simulink library "carnot"  (R2018b)
settings: Solver=VariableStepAuto  StartTime=0.0  StopTime=10.0  RelTol=1e-3
undefined symbols (not defined in the file or in its folder): A, A_earth, acol, Acol, ActPower1, ActPower2, ActPower3, Ad, Ad0, Ar, Au, Au0, Azimuth_Angle, B, Bd, Bd0, Br, Bu, Bu0, C, c1, c2, c3, c33, c4, c5, c6, CarnotCallbacks_Density, CarnotCallbacks_Enthalpy, CarnotCallbacks_Enthalpy2Temperature, CarnotCallbacks_Entropy, CarnotCallbacks_Evaporation_Enthalpy, CarnotCallbacks_GlobalMessageLevel, CarnotCallbacks_Grashof, CarnotCallbacks_Heat_Capacity, CarnotCallbacks_Kinematic_Viscosity, CarnotCallbacks_PMV_PPD, CarnotCallbacks_Prandtl, CarnotCallbacks_Saturation_Property, CarnotCallbacks_Saturation_Temperature, CarnotCallbacks_Saturation_Value_Water, CarnotCallbacks_Specific_Volume, CarnotCallbacks_Thermal_Conductivity, CarnotCallbacks_Vapour_Content, CarnotCallbacks_Vapour_Pressure, Cd, Cdl, Cr, Cu, Davies, Dd, DE_TRY2010_04_averageYear, delta_grd, density, DiameterLastPiece, dl, DPConstant, DPLinear, DPQuadratic, Dr ... (+59)
libraries: $bdroot x429, simulink x36, simulink_extras x12
(part 18 of 22)

== system carnot/Storage/Thermal/Storage_Ports ==
  Electric_Heating : Subsystem  mask(electric heating){hin=0.6, hout=0.65, nodes=nodes}
      mask prompts: hin "relative height start heating zone"; hout "relative height end heating zone"; nodes "Number of nodes (do not change here)"
      mask help: The block is an electric backup heating for the storage. Give inlet- and outlet-height as a relative position from 0 (= bottom) to 1 (= top).
      mask init:
      | hin = min(1, max(0, hin));
      | hout = min(1, max(0, hout));
      | 
      | if hin < hout
      |     inlet = max(ceil(hin*nodes),1);    % start node of heated zone
      |     outlet = max(ceil(hout*nodes),1);  % end node of heated zone
      | else
      |     outlet = max(ceil(hin*nodes),1);   % end node of heated zone
      |     inlet = max(ceil(hout*nodes),1);   % start node of heated zone
      | end
      | 
      | Q = zeros(nodes,1);                    % initilize power vector
      | if inlet < outlet
      |     Q(inlet:outlet) = ones(outlet-inlet+1,1); % set heated zone to One
      | else
      |     Q(outlet:inlet) = ones(inlet-outlet+1,1); % set heated zone to One
      | end
      | Q = Q./sum(Q);                         % sum over all elements must be one
      mask Help: web(fullfile(path_carnot('help'),'Electric_Heating.html'),'-helpbrowser')
      mask DialogControl ParameterTabVar0 Prompt: Geometry
      mask DialogControl ParameterTabVar01 Prompt: Top Mask Params
  HX_EN12977 : Subsystem  mask(heat exchanger for storage, data EN 12977){h_in=1, h_out=0, hgt=1, dia=0.03, height=-1, ua0=100, uam=0.1, uat=0.5, uat2=0, dplin=100, dpqua=100, nodes=nodes}
      mask prompts: h_in "relative height of inlet"; h_out "relative height of outlet"; hgt "Height of storage in m"; dia "Diameter of HX pipe [m]"; height "Height difference inlet-outlet [m]"; ua0 "uac: heat transfer coefficient [W/K /(kg/s) /(°C)]"; uam "uam: massflow dependent heat transfer [-]"; uat "uat: temperature dependent heat transfer [-]"; uat2 "uat2: temperature difference dependent heat transfer [-]"; dplin "Pressure drop coefficient dplin [Pa/(kg/s)]"; dpqua "Pressure drop coefficient dpqua [Pa/(kg/s)²]"; nodes "number of nodes"
      mask help:
      | The block transforms the incoming THV vector to a vector which the storage interprets as a heat exchanger.
      | Give inlet and outlet as a relative position 0=bottom to 1=top
      | The heat transfer is calculated by:
      | UA = uac * mdot^uam *
      |           ((Theatexchanger+Tstorage)/2)^uat *
      |           (Theatexchanger-Tstorage)^uat2
      mask init:
      | in = zeros(nodes,1);    % vector of length nodes
      | up = in;                % vector of length nodes
      | down = in;              % vector of length nodes
      | 
      | h_in = max(0,h_in);     % no nodes below 0
      | h_out = max(0,h_out);   % no nodes below 0
      | 
      | inlet = round(h_in*(nodes-1))+1;    % inlet position
      | outlet = round(h_out*(nodes-1))+1;  % outlet position
      | set_param(gcb,'height',num2str((h_out-h_in)*hgt));
      | % hgt = (h_out-h_in)*hgt;
      | 
      | in(inlet)=1;
      | 
      | if (h_in < h_out)           % if inlet below outlet
      |     up(inlet:outlet)=1;     % upwards
      | elseif (h_in > h_out)       % else if inlet above outlet
      |     down(outlet:inlet)=1;   % downwards
      | end
      mask Help: web(['file:///' fullfile(path_carnot('help'),'StoragePorts_HeatExchangerModels.html')],'-helpbrowser')
      mask TypeOptions dia: Pressure_Drop_StorageHX/dia
      mask TypeOptions height: Pressure_Drop_StorageHX/hgt
      mask TypeOptions ua0: sfun_storage_heatexchanger/p1
      mask TypeOptions uam: sfun_storage_heatexchanger/p2
      mask TypeOptions uat: sfun_storage_heatexchanger/p3
      mask TypeOptions uat2: sfun_storage_heatexchanger/p4
      mask TypeOptions dplin: Pressure_Drop_StorageHX/dplin
      mask TypeOptions dpqua: Pressure_Drop_StorageHX/dpqua
      mask TypeOptions nodes: sfun_storage_heatexchanger/nodes
      mask DialogControl ParameterTabVar0 Prompt: Geometry
      mask DialogControl ParameterTabVar01 Prompt: Heat transfer
      mask DialogControl ParameterTabVar012 Prompt: Pressure drop
      mask DialogControl ParameterTabVar0123 Prompt: Calculation
      mask Display: disp('HX EN12977')
  HX_EN12977_stratified : Subsystem  mask(stratified heat exchanger for storage, data EN 12977){h_in=1, h_out=0, hgt=height, dia=0.03, height=, ua0=100, uam=0.1, uat=0.5, uat2=0, dplin=100, dpqua=100, nodes=10}
      mask prompts: h_in "relative height of inlet"; h_out "relative height of outlet"; hgt "Height of storage in m"; dia "Diameter of HX pipe [m]"; height "Height difference inlet-outlet [m]"; ua0 "uac: heat transfer coefficient [W/K /(kg/s) /(°C)]"; uam "uam: massflow dependent heat transfer [-]"; uat "uat: temperature dependent heat transfer [-]"; uat2 "uat2: temperature difference dependent heat transfer [-]"; dplin "Pressure drop coefficient dplin [Pa/(kg/s)]"; dpqua "Pressure drop coefficient dpqua [Pa/(kg/s)²]"; nodes "number of nodes"
      mask help:
      | The block transforms the incoming THV vector to a vector which the storage interprets as a heat exchanger.
      | Give inlet and outlet as a relative position 0=bottom to 1=top
      | The heat transfer is calculated by:
      | UA = uac * mdot^uam *
      |           ((Theatexchanger+Tstorage)/2)^uat *
      |           (Theatexchanger-Tstorage)^uat2
      | Stratified:
      | For charging (inlet above outlet) the heat transfer starts when the storage temperature is below the heat exchanger temperature.
      | For discharging (outlet above inlet) the heat transfer starts when the storage temperature is above the heat exchanger temperature.
      mask init: same as carnot/Storage/Thermal/Storage_Ports/HX_EN12977
      mask Help: web(['file:///' fullfile(path_carnot('help'),'StoragePorts_HeatExchangerModels.html')],'-helpbrowser')
      mask TypeOptions dia: Pressure_Drop_StorageHX/dia
      mask TypeOptions height: Pressure_Drop_StorageHX/hgt
      mask TypeOptions ua0: sfun_storage_heatexchanger/p1
      mask TypeOptions uam: sfun_storage_heatexchanger/p2
      mask TypeOptions uat: sfun_storage_heatexchanger/p3
      mask TypeOptions uat2: sfun_storage_heatexchanger/p4
      mask TypeOptions dplin: Pressure_Drop_StorageHX/dplin
      mask TypeOptions dpqua: Pressure_Drop_StorageHX/dpqua
      mask TypeOptions nodes: sfun_storage_heatexchanger/nodes
      mask DialogControl ParameterTabVar0 Prompt: Geometry
      mask DialogControl ParameterTabVar01 Prompt: Heat transfer
      mask DialogControl ParameterTabVar012 Prompt: Pressure drop
      mask DialogControl ParameterTabVar0123 Prompt: Calculation
      mask Display: disp('HX EN12977 STRAT')
  HX_data_fit : Subsystem  mask(heat exchanger for storage, fitted data){h_in=1, h_out=0, hgt=1, dia=0.03, height=-1, ua0=100, uam=0, uat=0, dplin=10, dpqua=10, nodes=10}
      mask prompts: h_in "relative height of inlet"; h_out "relative height of outlet"; hgt "Height of storage in m"; dia "Diameter of HX pipe [m]"; height "Height difference inlet-outlet [m]"; ua0 "uac: constant heat transfer coefficient [W/K]"; uam "uam: massflow dependent heat transfer [W*s/(K*kg)]"; uat "uat: temperature difference dependent heat transfer [W/K²]"; dplin "Pressure drop coefficient dplin [Pa/(kg/s)]"; dpqua "Pressure drop coefficient dpqua [Pa/(kg/s)²]"; nodes "Number of nodes"
      mask help:
      | The block transforms the incoming THV vector to a vector which the storage interprets as a heat exchanger.
      | Give inlet and outlet as a relative position 0=bottom to 1=top
      | The heat transfer is calculated by:
      | UA = uac + mdot*uam + (Theatexchanger-Tstorage)*uat
      mask init:
      | in = zeros(nodes,1);    % vector of length nodes
      | up = in;                % vector of length nodes
      | down = in;              % vector of length nodes
      | 
      | h_in = max(0,h_in);     % no nodes below 0
      | h_out = max(0,h_out);   % no nodes below 0
      | 
      | inlet = round(h_in*(nodes-1))+1;    % inlet position
      | outlet = round(h_out*(nodes-1))+1;  % outlet position
      | set_param(gcb,'height',num2str((h_out-h_in)*hgt));
      | in(inlet)=1;
      | 
      | if (h_in < h_out)           % if inlet below outlet
      |     up(inlet:outlet)=1;     % upwards
      | elseif (h_in > h_out)       % else if inlet above outlet
      |     down(outlet:inlet)=1;   % downwards
      | end
      mask Help: web(fullfile(path_carnot('help'),'StoragePorts_HeatExchangerModels.html'),'-helpbrowser')
      mask TypeOptions dia: Pressure_Drop_StorageHX/dia
      mask TypeOptions height: Pressure_Drop_StorageHX/hgt
      mask TypeOptions ua0: sfun_storage_heatexchanger/p1
      mask TypeOptions uam: sfun_storage_heatexchanger/p2
      mask TypeOptions uat: sfun_storage_heatexchanger/p3
      mask TypeOptions dplin: Pressure_Drop_StorageHX/dplin
      mask TypeOptions dpqua: Pressure_Drop_StorageHX/dpqua
      mask TypeOptions nodes: sfun_storage_heatexchanger/nodes
      mask DialogControl ParameterTabVar0 Prompt: Geometry
      mask DialogControl ParameterTabVar01 Prompt: Heat transfer
      mask DialogControl ParameterTabVar012 Prompt: Pressure drop
      mask DialogControl ParameterTabVar0123 Prompt: Calculation
      mask Display: disp('HX data')
  HX_data_fit_stratified : Subsystem  mask(stratified heat exchanger for storage, fitted data){h_in=1, h_out=0, hgt=1.5, dia=0.03, height=-1.5, ua0=800, uam=0, uat=0, dplin=100, dpqua=100, nodes=10}
      mask prompts: h_in "relative height of inlet"; h_out "relative height of outlet"; hgt "Height of storage in m"; dia "Diameter of HX pipe [m]"; height "Height difference inlet-outlet [m]"; ua0 "uac: constant heat transfer coefficient [W/K]"; uam "uam: massflow dependent heat transfer [W*s/(K*kg)]"; uat "uat: temperature difference dependent heat transfer [W/K²]"; dplin "Pressure drop coefficient dplin [Pa/(kg/s)]"; dpqua "Pressure drop coefficient dpqua [Pa/(kg/s)²]"; nodes "number of nodes"
      mask help:
      | The block transforms the incoming THV vector to a vector which the storage interprets as a heat exchanger.
      | Give inlet and outlet as a relative position 0=bottom to 1=top
      | The heat transfer is calculated by:
      | UA = uac + mdot*uam + (Theatexchanger-Tstorage)*uat
      |
      | Stratified:
      | For charging (inlet above outlet) the heat transfer starts when the storage temperature is below the heat exchanger temperature.
      | For discharging (outlet above inlet) the heat transfer starts when the storage temperature is above the heat exchanger temperature.
      mask init: same as carnot/Storage/Thermal/Storage_Ports/HX_EN12977
      mask Help: web(['file:///' fullfile(path_carnot('help'),'StoragePorts_HeatExchangerModels.html')],'-helpbrowser')
      mask TypeOptions dia: Pressure_Drop_StorageHX/dia
      mask TypeOptions height: Pressure_Drop_StorageHX/hgt
      mask TypeOptions ua0: sfun_storage_heatexchanger/p1
      mask TypeOptions uam: sfun_storage_heatexchanger/p2
      mask TypeOptions uat: sfun_storage_heatexchanger/p3
      mask TypeOptions dplin: Pressure_Drop_StorageHX/dplin
      mask TypeOptions dpqua: Pressure_Drop_StorageHX/dpqua
      mask TypeOptions nodes: sfun_storage_heatexchanger/nodes
      mask DialogControl ParameterTabVar0 Prompt: Geometry
      mask DialogControl ParameterTabVar01 Prompt: Heat transfer
      mask DialogControl ParameterTabVar012 Prompt: Pressure drop
      mask DialogControl ParameterTabVar0123 Prompt: Calculation
      mask Display: disp('HX data STRAT')
  HX_finned_tube : Subsystem  mask(finned tube heat exchanger for storage){h_in=0.5, h_out=0, hgt=1, dpipe=0.03, swall=0.001, lpipe=10, cond=50, dfin=0.05, sfin=0.002, nfin=100, height=-0.5, dplin=100, dpqua=100, nodes=10}
      mask prompts: h_in "relative height of inlet"; h_out "relative height of outlet"; hgt "Height of storage in m"; dpipe "outer diameter of HX pipe in m (without fins)"; swall "thickness of pipe wall in m"; lpipe "length of HX pipe in m"; cond "thermal conductivity of HX wall in W/m/K"; dfin "diameter of HX pipe with fins in m"; sfin "wall thickness of fins in m"; nfin "number of fins per length in 1/m"; height "Height difference inlet-outlet [m]"; dplin "Pressure drop coefficient dplin [Pa/(kg/s)]"; dpqua "Pressure drop coefficient dpqua [Pa/(kg/s)²]"; nodes "number of nodes"
      mask help:
      | The block transforms the incoming THV vector to a vector which the storage interprets as a heat exchanger.
      | Give inlet and outlet as a relative position 0=bottom to 1=top
      | The heat transfer is calculated by a theoretical equation from Wagner: Waermeuebertragung, Vogel Fachbuch, 1991
      mask init:
      | in = zeros(nodes,1);    % vector of length nodes
      | up = in;                % vector of length nodes
      | down = in;              % vector of length nodes
      | 
      | h_in = max(0,h_in);     % no nodes below 0
      | h_out = max(0,h_out);   % no nodes below 0
      | set_param(gcb,'height',num2str((h_out-h_in)*hgt));
      | % hgt = (h_out-h_in)*hgt;
      | 
      | inlet = round(h_in*(nodes-1))+1;    % inlet position
      | outlet = round(h_out*(nodes-1))+1;  % outlet position
      | 
      | in(inlet)=1;
      | 
      | if (h_in < h_out)           % if inlet below outlet
      |     up(inlet:outlet)=1;     % upwards
      | elseif (h_in > h_out)       % else if inlet above outlet
      |     down(outlet:inlet)=1;   % downwards
      | end
      | 
      | dfin = max(dfin,dpipe);
      | nfin = max(nfin, 0);
      | if (sfin < 1e-5)
      |    sfin = 1e-5;
      |    disp('fin width set to minimum 0.01 mm')
      | end
      mask Help: web(['file:///' fullfile(path_carnot('help'),'StoragePorts_HeatExchangerModels.html')],'-helpbrowser')
      mask TypeOptions dpipe: sfun_storage_heatexchanger/p1 | Pressure_Drop_StorageHX/dia
      mask TypeOptions swall: sfun_storage_heatexchanger/p2
      mask TypeOptions lpipe: sfun_storage_heatexchanger/p3
      mask TypeOptions cond: sfun_storage_heatexchanger/p4
      mask TypeOptions dfin: sfun_storage_heatexchanger/p5
      mask TypeOptions sfin: sfun_storage_heatexchanger/p6
      mask TypeOptions nfin: sfun_storage_heatexchanger/p7
      mask TypeOptions height: Pressure_Drop_StorageHX/hgt
      mask TypeOptions dplin: Pressure_Drop_StorageHX/dplin
      mask TypeOptions dpqua: Pressure_Drop_StorageHX/dpqua
      mask TypeOptions nodes: sfun_storage_heatexchanger/nodes
      mask DialogControl ParameterTabVar0 Prompt: Heat Exchanger
      mask DialogControl ParameterTabVar01 Prompt: Pressure drop
      mask DialogControl ParameterTabVar012 Prompt: Calculation
      mask Display: disp('HX finned tube')
  HX_finned_tube_stratified : Subsystem  mask(finned tube heat exchanger for storage){h_in=1, h_out=0, hgt=1, dpipe=0.03, swall=0.001, lpipe=10, cond=50, dfin=0.05, sfin=0.002, nfin=100, height=-1, dplin=100, dpqua=100, nodes=10}
      mask prompts: h_in "relative height of inlet"; h_out "relative height of outlet"; hgt "Height of storage in m"; dpipe "outer diameter of HX pipe in m (without fins)"; swall "thickness of pipe wall in m"; lpipe "length of HX pipe in m"; cond "thermal conductivity of HX wall in W/m/K"; dfin "diameter of HX pipe with fins in m"; sfin "wall thickness of fins in m"; nfin "number of fins per length in 1/m"; height "Height difference inlet-outlet [m]"; dplin "Pressure drop coefficient dplin [Pa/(kg/s)]"; dpqua "Pressure drop coefficient dpqua [Pa/(kg/s)²]"; nodes "number of nodes"
      mask help:
      | The block transforms the incoming THV vector to a vector which the storage interprets as a heat exchanger.
      | Give inlet and outlet as a relative position 0=bottom to 1=top
      | The heat transfer is calculated by a theoretical equation from Wagner: Waermeuebertragung, Vogel Fachbuch, 1991
      mask init: same as carnot/Storage/Thermal/Storage_Ports/HX_finned_tube
      mask Help: web(['file:///' fullfile(path_carnot('help'),'StoragePorts_HeatExchangerModels.html')],'-helpbrowser')
      mask TypeOptions dpipe: sfun_storage_heatexchanger/p1 | Pressure_Drop_StorageHX/dia
      mask TypeOptions swall: sfun_storage_heatexchanger/p2
      mask TypeOptions lpipe: sfun_storage_heatexchanger/p3
      mask TypeOptions cond: sfun_storage_heatexchanger/p4
      mask TypeOptions dfin: sfun_storage_heatexchanger/p5
      mask TypeOptions sfin: sfun_storage_heatexchanger/p6
      mask TypeOptions nfin: sfun_storage_heatexchanger/p7
      mask TypeOptions height: Pressure_Drop_StorageHX/hgt
      mask TypeOptions dplin: Pressure_Drop_StorageHX/dplin
      mask TypeOptions dpqua: Pressure_Drop_StorageHX/dpqua
      mask TypeOptions nodes: sfun_storage_heatexchanger/nodes
      mask DialogControl ParameterTabVar0 Prompt: Heat Exchanger
      mask DialogControl ParameterTabVar01 Prompt: Pressure drop
      mask DialogControl ParameterTabVar012 Prompt: Calculation
      mask Display: disp('HX finned tube STRAT')
  HX_tube : Subsystem  mask(smooth tube heat exchanger for storage){h_in=0.5, h_out=0, hgt=1.5, dpipe=0.03, swall=0.001, lpipe=10, cond=50, height=-0.75, dplin=100, dpqua=100, nodes=10}
      mask prompts: h_in "relative height of inlet"; h_out "relative height of outlet"; hgt "Height of storage in m"; dpipe "outer diameter of HX pipe in m"; swall "thickness of pipe wall in m"; lpipe "length of HX pipe in m"; cond "thermal conductivity of HX wall in W/m/K"; height "Height difference inlet-outlet [m]"; dplin "Pressure drop coefficient dplin [Pa/(kg/s)]"; dpqua "Pressure drop coefficient dpqua [Pa/(kg/s)²]"; nodes "number of nodes"
      mask help:
      | The block transforms the incoming THV vector to a vector which the storage interprets as a heat exchanger.
      | Give inlet and outlet as a relative position 0=bottom to 1=top
      | The heat transfer is calculated with an equation from Wagner: Waermeuebertragung, Vogel-Verlag, 1991
      mask init: same as carnot/Storage/Thermal/Storage_Ports/HX_EN12977
      mask Help: web(['file:///' fullfile(path_carnot('help'),'StoragePorts_HeatExchangerModels.html')],'-helpbrowser')
      mask TypeOptions dpipe: sfun_storage_heatexchanger/p1
      mask TypeOptions swall: sfun_storage_heatexchanger/p2
      mask TypeOptions lpipe: sfun_storage_heatexchanger/p3
      mask TypeOptions cond: sfun_storage_heatexchanger/p4
      mask TypeOptions height: Pressure_Drop_StorageHX/hgt
      mask TypeOptions dplin: Pressure_Drop_StorageHX/dplin
      mask TypeOptions dpqua: Pressure_Drop_StorageHX/dpqua
      mask TypeOptions nodes: sfun_storage_heatexchanger/nodes
      mask DialogControl ParameterTabVar0 Prompt: Heat Exchanger
      mask DialogControl ParameterTabVar01 Prompt: Pressure drop
      mask DialogControl ParameterTabVar012 Prompt: Calculation
      mask Display: disp('HX tube')
  HX_tube_stratified : Subsystem  mask(smooth tube heat exchanger for storage){h_in=1, h_out=0, hgt=1.5, dpipe=0.03, swall=0.001, lpipe=10, cond=50, height=-1.5, dplin=100, dpqua=100, nodes=10}
      mask prompts: h_in "relative height of inlet"; h_out "relative height of outlet"; hgt "Height of storage in m"; dpipe "outer diameter of HX pipe in m"; swall "thickness of pipe wall in m"; lpipe "length of HX pipe in m"; cond "thermal conductivity of HX wall in W/m/K"; height "Height difference inlet-outlet [m]"; dplin "Pressure drop coefficient dplin [Pa/(kg/s)]"; dpqua "Pressure drop coefficient dpqua [Pa/(kg/s)²]"; nodes "number of nodes"
      mask help:
      | The block transforms the incoming THV vector to a vector which the storage interprets as a heat exchanger.
      | Give inlet and outlet as a relative position 0=bottom to 1=top
      | The heat transfer is calculated with an equation from Wagner: Waermeuebertragung, Vogel-Verlag, 1991
      mask init: same as carnot/Storage/Thermal/Storage_Ports/HX_EN12977
      mask Help: web(['file:///' fullfile(path_carnot('help'),'StoragePorts_HeatExchangerModels.html')],'-helpbrowser')
      mask TypeOptions dpipe: sfun_storage_heatexchanger/p1
      mask TypeOptions swall: sfun_storage_heatexchanger/p2
      mask TypeOptions lpipe: sfun_storage_heatexchanger/p3
      mask TypeOptions cond: sfun_storage_heatexchanger/p4
      mask TypeOptions height: Pressure_Drop_StorageHX/hgt
      mask TypeOptions dplin: Pressure_Drop_StorageHX/dplin
      mask TypeOptions dpqua: Pressure_Drop_StorageHX/dpqua
      mask TypeOptions nodes: sfun_storage_heatexchanger/nodes
      mask DialogControl ParameterTabVar0 Prompt: Heat Exchanger
      mask DialogControl ParameterTabVar01 Prompt: Pressure drop
      mask DialogControl ParameterTabVar012 Prompt: Calculation
      mask Display: disp('HX tube STRAT')
  Pipe_Connection : Subsystem  mask(pipe connection to storage){h_in=0, h_out=1, hgt=1, dpipe=0.03, dstg=1, height=1, nodes=nodes}
      mask prompts: h_in "relative height of inlet, range from 0 (= bottom) to 1 (= top)"; h_out "relative height of outlet, range from 0 (= bottom) to 1 (= top)"; hgt "Height of storage in m"; dpipe "Diameter of pipe in m"; dstg "Diameter of storage in m"; height "Height difference inlet-outlet"; nodes "Number of nodes of storage"
      mask help: The block transforms the incoming THV vector to a vector which the storage interprets as a flow into the storage fluid.
      mask init:
      | in = zeros(nodes,1);    % vector of length nodes
      | up = in;                % vector of length nodes
      | down = in;              % vector of length nodes
      | 
      | h_in = max(0,min(h_in,1));     % no nodes below 0
      | h_out = max(0,min(h_out,1));   % no nodes below 0
      | set_param(gcb,'height',num2str((h_out-h_in)*hgt));
      |  
      | inlet = max(ceil(h_in*nodes),1);    % inlet position
      | outlet = max(ceil(h_out*nodes),1);  % outlet position
      |  
      | in(inlet)=1;
      |  
      | idx_in_out = inlet:outlet;
      | if (inlet < outlet)         % if inlet below outlet
      |     up(inlet:outlet-1)=1;   % upwards
      | elseif (inlet > outlet)     % else if inlet above outlet
      |     down(outlet:inlet-1)=1; % downwards
      |     idx_in_out = outlet:inlet;
      | end
      mask Help: web(fullfile(path_carnot('help'),'StoragePorts_PipeConnections.html'),'-helpbrowser')
      mask TypeOptions dpipe: Pressure_Drop_StoragePipe/dpipe
      mask TypeOptions dstg: Pressure_Drop_StoragePipe/dstg
      mask TypeOptions height: Pressure_Drop_StoragePipe/hgt
      mask DialogControl ParameterTabVar0 Prompt: Geometry
      mask DialogControl ParameterTabVar02 Prompt: Calulation
      mask Display: disp('Pipe')
  Pipe_stratified : Subsystem  mask(pipe connection to storage){h_in=0, h_out=1, hgt=1, dpipe=0.02, dstg=1, height=1, nodes=nodes}
      mask prompts: h_in "relative height of inlet"; h_out "relative height of outlet"; hgt "Height of storage in m"; dpipe "Diameter of pipe in m"; dstg "Diameter of storage in m"; height "Height difference inlet-outlet"; nodes "Number of nodes"
      mask help:
      | The block transforms the incoming THV vector to a vector which the storage interprets as a flow into the storage fluid.
      | Give inlet- and outlet-height as a relative position from 0 (= bottom) to 1 (= top).
      mask init:
      | in = zeros(nodes,1);    % vector of length nodes
      | up = in;                % vector of length nodes
      | down = in;              % vector of length nodes
      | h_in = max(0,min(h_in,1));     % no nodes below 0 and above 1
      | h_out = max(0,min(h_out,1));   % no nodes below 0 and above 1
      | set_param(gcb,'height',num2str((h_out-h_in)*hgt));
      | inlet = max(ceil(h_in*nodes),1);    % inlet position
      | outlet = max(ceil(h_out*nodes),1);  % outlet position
      | hgt = (h_out-h_in)*hgt;
      | in(inlet) = 1;
      | idx_in_out = inlet:outlet;
      | n_concerned = idx_in_out;
      | flowdir = 1;
      | if (inlet < outlet)             % if inlet below outlet
      |     up(inlet:outlet-1)=1;       % upwards
      | elseif (inlet > outlet)         % else if inlet above outlet
      |     down(outlet:inlet-1)=1;     % downwards
      |     idx_in_out = outlet:inlet;
      |     n_concerned = idx_in_out;
      |     flowdir = -1;
      | end
      mask Help: web(fullfile(path_carnot('help'),'StoragePorts_PipeConnections.html'),'-helpbrowser')
      mask TypeOptions dpipe: Pressure_Drop_StoragePipe/dpipe
      mask TypeOptions dstg: Pressure_Drop_StoragePipe/dstg
      mask TypeOptions height: Pressure_Drop_StoragePipe/hgt
      mask DialogControl ParameterTabVar0 Prompt: Geometry
      mask DialogControl ParameterTabVar02 Prompt: Calculation
      mask Display: disp('Pipe STRAT')

== system carnot/Storage/Thermal/Storage_Type_0 ==
  note: charging pipe connection
  Tamb : Inport
  THB_chg : Inport  Port=2
  Pel : Inport  Port=3
  Constant_THB : $bdroot/Source/Simple/Constant_THB  t=20  mdot=0  p=1e5  mID=No Pressure Drop  fluid=Water  mix=0  mix2=0  mix3=0  dia=0.02  hgt=0
  CreateSdat : $bdroot/Basic/Thermal_Models/CreateSdat  volume=volume  stgtype=stgtype
  Electric_Heating_1 : $bdroot/Storage/Thermal/Storage_Ports/Electric_Heating  hin=heater1start  hout=heater1end  nodes=nodes
  Pipe_Connection_1 : $bdroot/Storage/Thermal/Storage_Ports/Pipe_Connection  h_in=pipe1inlet  h_out=pipe1outlet  hgt=hgt  dpipe=pipe1dia  dstg=dia  height=-1.5279  nodes=nodes
  T_Sensor_Surface : $bdroot/Control/T_Sensor_Surface  pos=Tsensor  tdel=10  t0=mean(tini)
  select_T : Selector  InputPortWidth=nodes  IndexOptions=Index vector (dialog)  Indices=[1 2 3 4 5 6 7 8 9 10]  OutputSizes=1
  sfun_storageTnodes : $bdroot/Basic/Thermal_Models/sfun_storageTnodes  uloss=uwall  ubot=ubot  utop=utop  cond=axcond  volume=volume  dia=dia  standing=standing cylinder  tini=tini  nodes=nodes  nconnect=2  elimthermocline=2  condinvtc=1e5
  Sdat : Outport
  Tsensors : Outport  Port=2
  THBchg : Outport  Port=3
  wires:
  Electric_Heating_1/1 -> sfun_storageTnodes/3
  THB_chg/1 -> Pipe_Connection_1/2, CreateSdat/4, Electric_Heating_1/2  "THBinPipe2"
  Pel/1 -> CreateSdat/20, Electric_Heating_1/1  "PelHeater1"
  Constant_THB/1 -> CreateSdat/19, CreateSdat/18, CreateSdat/17, CreateSdat/16, CreateSdat/15, CreateSdat/6, CreateSdat/7, CreateSdat/8, CreateSdat/9, CreateSdat/10, CreateSdat/11, CreateSdat/12, CreateSdat/13, CreateSdat/14
  sfun_storageTnodes/1 -> CreateSdat/2  "Energy"
  Tamb/1 -> sfun_storageTnodes/1, CreateSdat/1  "Tamb"
  select_T/1 -> CreateSdat/3  "Tnodes"
  sfun_storageTnodes/2 -> select_T/1, T_Sensor_Surface/1, Pipe_Connection_1/1  "Tnodes"
  CreateSdat/1 -> Sdat/1
  Pipe_Connection_1/2 -> THBchg/1, CreateSdat/5  "THBoutPipe1"
  Pipe_Connection_1/1 -> sfun_storageTnodes/2
  T_Sensor_Surface/1 -> Tsensors/1

== system carnot/Storage/Thermal/Storage_Type_1 ==
  note: charging pipe connection
  note: discharging pipe connection
  Tamb : Inport
  THB_chg : Inport  Port=2
  THB_dis : Inport  Port=3
  Pel : Inport  Port=4
  Constant_THB : $bdroot/Source/Simple/Constant_THB  t=20  mdot=0  p=1e5  mID=No Pressure Drop  fluid=Water  mix=0  mix2=0  mix3=0  dia=0.02  hgt=0
  CreateSdat : $bdroot/Basic/Thermal_Models/CreateSdat  volume=volume  stgtype=stgtype
  Electric_Heating_1 : $bdroot/Storage/Thermal/Storage_Ports/Electric_Heating  hin=heater1start  hout=heater1end  nodes=nodes
  Pipe_Connection_1 : $bdroot/Storage/Thermal/Storage_Ports/Pipe_Connection  h_in=pipe1inlet  h_out=pipe1outlet  hgt=hgt  dpipe=pipe1dia  dstg=dia  height=-1.7684  nodes=nodes
  Pipe_Connection_2 : $bdroot/Storage/Thermal/Storage_Ports/Pipe_Connection  h_in=pipe2inlet  h_out=pipe2outlet  hgt=hgt  dpipe=pipe2dia  dstg=dia  height=1.7684  nodes=nodes
  T_Sensor_Surface : $bdroot/Control/T_Sensor_Surface  pos=Tsensor  tdel=10  t0=mean(tini)
  select_T : Selector  InputPortWidth=nodes  IndexOptions=Index vector (dialog)  Indices=[1 2 3 4 5 6 7 8 9 10]  OutputSizes=1
  sfun_storageTnodes : $bdroot/Basic/Thermal_Models/sfun_storageTnodes  uloss=uwall  ubot=ubot  utop=utop  cond=axcond  volume=volume  dia=dia  standing=standing cylinder  tini=tini  nodes=nodes  nconnect=3  elimthermocline=2  condinvtc=1e5
  Sdat : Outport
  Tsensors : Outport  Port=2
  THBchg : Outport  Port=3
  THBdis : Outport  Port=4
  wires:
  Electric_Heating_1/1 -> sfun_storageTnodes/4
  THB_dis/1 -> Pipe_Connection_2/2, CreateSdat/6, Electric_Heating_1/2  "THBinPipe2"
  Pel/1 -> CreateSdat/20, Electric_Heating_1/1  "PelHeater1"
  sfun_storageTnodes/1 -> CreateSdat/2  "Energy"
  Pipe_Connection_2/2 -> CreateSdat/7, THBdis/1  "THBoutPipe2"
  Pipe_Connection_2/1 -> sfun_storageTnodes/3
  Tamb/1 -> sfun_storageTnodes/1, CreateSdat/1  "Tamb"
  select_T/1 -> CreateSdat/3  "Tnodes"
  sfun_storageTnodes/2 -> select_T/1, T_Sensor_Surface/1, Pipe_Connection_2/1, Pipe_Connection_1/1  "Tnodes"
  CreateSdat/1 -> Sdat/1
  THB_chg/1 -> CreateSdat/4, Pipe_Connection_1/2  "THBinPipe1"
  Pipe_Connection_1/2 -> CreateSdat/5, THBchg/1  "THBoutPipe1"
  Pipe_Connection_1/1 -> sfun_storageTnodes/2
  T_Sensor_Surface/1 -> Tsensors/1
  Constant_THB/1 -> CreateSdat/16, CreateSdat/17, CreateSdat/18, CreateSdat/19, CreateSdat/15, CreateSdat/14, CreateSdat/13, CreateSdat/12, CreateSdat/11, CreateSdat/10, CreateSdat/9, CreateSdat/8

== system carnot/Storage/Thermal/Storage_Type_11 ==
  note: Buffer storage as a model of the T-piece
      | no thermal losses to ambient
  note: charging pipe connection
  note: discharging pipe connection
  Tamb : Inport
  THB_chg : Inport  Port=2
  THB_dis : Inport  Port=3
  Pel : Inport  Port=4
  Add : Sum
  Bus Selector : BusSelector  OutputSignals=energy
  Constant : Constant  Value=10
  Constant_THB : $bdroot/Source/Simple/Constant_THB  t=20  mdot=0  p=1e5  mID=No Pressure Drop  fluid=Water  mix=0  mix2=0  mix3=0  dia=0.02  hgt=0
  CreateSdat : $bdroot/Basic/Thermal_Models/CreateSdat  volume=volume  stgtype=stgtype
  Electric_Heating_1 : $bdroot/Storage/Thermal/Storage_Ports/Electric_Heating  hin=heater1start  hout=heater1end  nodes=nodes
  Ground : Ground
  Pipe with T-piece : $bdroot/Storage/Thermal/Storage_Type_1  t0=10  hgt=0.5093  stgtype=1  tini=10  mpts=1  PathName=fullfile(path_carnot('libsl'),'Storage','Thermal','Storage_Type_11','parameter_set')  FileName='<user defined>'  userPath=off  userParam=on  uwall=0  ubot=0  utop=0  axcond=0  volume=0.004  dia=0.1  standing=standing cylinder  nodes=1  mpoints=1  Tsensor=0.5  pipe1inlet=1  pipe1outlet=0  pipe1dia=0.03  pipe2inlet=0  pipe2outlet=1  pipe2dia=0.03  heater1start=0.6  heater1end=0.65
  Pipe_Connection_1 : $bdroot/Storage/Thermal/Storage_Ports/Pipe_Connection  h_in=pipe1inlet  h_out=pipe1outlet  hgt=hgt  dpipe=pipe1dia  dstg=dia  height=-1.7684  nodes=nodes
  Pipe_Connection_2 : $bdroot/Storage/Thermal/Storage_Ports/Pipe_Connection  h_in=pipe2inlet  h_out=pipe2outlet  hgt=hgt  dpipe=pipe2dia  dstg=dia  height=1.5916  nodes=nodes
  T_Sensor_Surface : $bdroot/Control/T_Sensor_Surface  pos=Tsensor  tdel=10  t0=mean(tini)
  Terminator : Terminator
  select_T : Selector  InputPortWidth=nodes  IndexOptions=Index vector (dialog)  Indices=[1 2 3 4 5 6 7 8 9 10]  OutputSizes=1
  sfun_storageTnodes : $bdroot/Basic/Thermal_Models/sfun_storageTnodes  uloss=uwall  ubot=ubot  utop=utop  cond=axcond  volume=volume  dia=dia  standing=standing cylinder  tini=tini  nodes=nodes  nconnect=3  elimthermocline=2  condinvtc=1e5
  Sdat : Outport
  Tsensors : Outport  Port=2
  THBchg : Outport  Port=3
  THBdis : Outport  Port=4
  wires:
  Ground/1 -> Pipe with T-piece/4
  Electric_Heating_1/1 -> sfun_storageTnodes/4
  THB_dis/1 -> CreateSdat/6, Pipe_Connection_2/2, Electric_Heating_1/2  "THBinPipe2"
  Pel/1 -> CreateSdat/20, Electric_Heating_1/1  "PelHeater1"
  Bus Selector/1 -> Add/1  "<energy>"
  Add/1 -> CreateSdat/2
  Pipe_Connection_2/2 -> Pipe with T-piece/3  "THBoutPipe2"
  Pipe_Connection_1/2 -> CreateSdat/5, THBchg/1  "THBoutPipe1"
  Pipe with T-piece/4 -> THBdis/1, CreateSdat/7  "THBoutPipe2"
  THB_chg/1 -> CreateSdat/4, Pipe with T-piece/2  "THBinPipe1"
  sfun_storageTnodes/1 -> Add/2  "Energy"
  Pipe_Connection_2/1 -> sfun_storageTnodes/3
  Tamb/1 -> sfun_storageTnodes/1, CreateSdat/1  "Tamb"
  select_T/1 -> CreateSdat/3  "Tnodes"
  sfun_storageTnodes/2 -> select_T/1, T_Sensor_Surface/1, Pipe_Connection_1/1, Pipe_Connection_2/1  "Tnodes"
  CreateSdat/1 -> Sdat/1
  Pipe_Connection_1/1 -> sfun_storageTnodes/2
  T_Sensor_Surface/1 -> Tsensors/1
  Constant_THB/1 -> CreateSdat/16, CreateSdat/17, CreateSdat/18, CreateSdat/19, CreateSdat/15, CreateSdat/14, CreateSdat/13, CreateSdat/12, CreateSdat/11, CreateSdat/10, CreateSdat/9, CreateSdat/8
  Constant/1 -> Pipe with T-piece/1
  Pipe with T-piece/2 -> Terminator/1
  Pipe with T-piece/1 -> Bus Selector/1
  Pipe with T-piece/3 -> Pipe_Connection_1/2

== system carnot/Storage/Thermal/Storage_Type_12 ==
  note: Elecric heater uses a THB of
      | a pipe connection for the fluid
      | type informations.
  note: charging pipe connection
  note: discharging pipe connection
  note: charging pipe connection
  note: discharging pipe connection
  Tamb : Inport
  THB_chg1 : Inport  Port=2
  THB_chg2 : Inport  Port=3
  THB_dis1 : Inport  Port=4
  THB_dis2 : Inport  Port=5
  Pel : Inport  Port=6
  Constant_THB : $bdroot/Source/Simple/Constant_THB  t=20  mdot=0  p=1e5  mID=No Pressure Drop  fluid=Water  mix=0  mix2=0  mix3=0  dia=0.02  hgt=0
  CreateSdat : $bdroot/Basic/Thermal_Models/CreateSdat  volume=volume  stgtype=stgtype
  Electric_Heating_1 : $bdroot/Storage/Thermal/Storage_Ports/Electric_Heating  hin=heater1start  hout=heater1end  nodes=nodes
  Pipe_Connection_1 : $bdroot/Storage/Thermal/Storage_Ports/Pipe_Connection  h_in=pipe1inlet  h_out=pipe1outlet  hgt=hgt  dpipe=pipe1dia  dstg=dia  height=-1.7684  nodes=nodes
  Pipe_Connection_2 : $bdroot/Storage/Thermal/Storage_Ports/Pipe_Connection  h_in=pipe2inlet  h_out=pipe2outlet  hgt=hgt  dpipe=pipe2dia  dstg=dia  height=-1.7684  nodes=nodes
  Pipe_Connection_3 : $bdroot/Storage/Thermal/Storage_Ports/Pipe_Connection  h_in=pipe3inlet  h_out=pipe3outlet  hgt=hgt  dpipe=pipe3dia  dstg=dia  height=1.7684  nodes=nodes
  Pipe_Connection_4 : $bdroot/Storage/Thermal/Storage_Ports/Pipe_Connection  h_in=pipe4inlet  h_out=pipe4outlet  hgt=hgt  dpipe=pipe4dia  dstg=dia  height=1.7684  nodes=nodes
  T_Sensor_Surface : $bdroot/Control/T_Sensor_Surface  pos=Tsensor  tdel=10  t0=mean(tini)
  select_T : Selector  InputPortWidth=nodes  IndexOptions=Index vector (dialog)  Indices=[1 2 3 4 5 6 7 8 9 10]  OutputSizes=1
  sfun_storageTnodes : $bdroot/Basic/Thermal_Models/sfun_storageTnodes  uloss=uwall  ubot=ubot  utop=utop  cond=axcond  volume=volume  dia=dia  standing=standing cylinder  tini=tini  nodes=nodes  nconnect=5  elimthermocline=2  condinvtc=1e5
  Sdat : Outport
  Tsensors : Outport  Port=2
  THBchg1 : Outport  Port=3
  THBchg2 : Outport  Port=4
  THBdis1 : Outport  Port=5
  THBdis2 : Outport  Port=6
  wires:
  CreateSdat/1 -> Sdat/1
  Pipe_Connection_2/1 -> sfun_storageTnodes/3
  Pipe_Connection_2/2 -> CreateSdat/7, THBchg2/1  "THBoutPipe2"
  THB_chg2/1 -> CreateSdat/6, Pipe_Connection_2/2  "THBinPipe2"
  sfun_storageTnodes/2 -> T_Sensor_Surface/1, select_T/1, Pipe_Connection_2/1, Pipe_Connection_3/1, Pipe_Connection_4/1, Pipe_Connection_1/1  "Tnodes"
  Pipe_Connection_4/1 -> sfun_storageTnodes/5
  Pipe_Connection_4/2 -> CreateSdat/11, THBdis2/1  "THBoutPipe4"
  THB_dis2/1 -> CreateSdat/10, Pipe_Connection_4/2, Electric_Heating_1/2  "THBinPipe4"
  Electric_Heating_1/1 -> sfun_storageTnodes/6
  THB_dis1/1 -> CreateSdat/8, Pipe_Connection_3/2  "THBinPipe3"
  Pel/1 -> CreateSdat/20, Electric_Heating_1/1  "PelHeater1"
  sfun_storageTnodes/1 -> CreateSdat/2  "Energy"
  Pipe_Connection_3/2 -> CreateSdat/9, THBdis1/1  "THBoutPipe3"
  Pipe_Connection_3/1 -> sfun_storageTnodes/4
  Tamb/1 -> sfun_storageTnodes/1, CreateSdat/1  "Tamb"
  select_T/1 -> CreateSdat/3  "Tnodes"
  THB_chg1/1 -> CreateSdat/4, Pipe_Connection_1/2  "THBinPipe1"
  Pipe_Connection_1/2 -> CreateSdat/5, THBchg1/1  "THBoutPipe1"
  Pipe_Connection_1/1 -> sfun_storageTnodes/2
  T_Sensor_Surface/1 -> Tsensors/1
  Constant_THB/1 -> CreateSdat/17, CreateSdat/18, CreateSdat/19, CreateSdat/15, CreateSdat/14, CreateSdat/13, CreateSdat/12, CreateSdat/16

== system carnot/Storage/Thermal/Storage_Type_2 ==
  note: upper heat exchanger (backup heater)
  note: pipe connection for DHW
  note: pipe connection for DHW circulation
  Tamb : Inport
  THB_HX : Inport  Port=2
  THB_dhw : Inport  Port=3
  THB_circ : Inport  Port=4
  Pel : Inport  Port=5
  Constant_THB : $bdroot/Source/Simple/Constant_THB  t=20  mdot=0  p=1e5  mID=No Pressure Drop  fluid=Water  mix=0  mix2=0  mix3=0  dia=0.02  hgt=0
  Constant_THB1 : $bdroot/Source/Simple/Constant_THB  t=20  mdot=0  p=1e5  mID=No Pressure Drop  fluid=Water  mix=0  mix2=0  mix3=0  dia=0.02  hgt=0
  CreateSdat : $bdroot/Basic/Thermal_Models/CreateSdat  volume=1  stgtype=stgtype
  Electric_Heating_1 : $bdroot/Storage/Thermal/Storage_Ports/Electric_Heating  hin=heater1start  hout=heater1end  nodes=nodes
  HX_EN12977_1 : $bdroot/Storage/Thermal/Storage_Ports/HX_EN12977  h_in=hx1inlet  h_out=hx1outlet  hgt=hgt  dia=hx1dia  height=-0.75762  ua0=hx1uac  uam=hx1uam  uat=hx1uat  uat2=uat2  dplin=hx1dplin  dpqua=hx1dpqua  nodes=nodes
  Pipe_Connection_1 : $bdroot/Storage/Thermal/Storage_Ports/Pipe_Connection  h_in=pipe1inlet  h_out=pipe1outlet  hgt=hgt  dpipe=pipe1dia  dstg=dia  height=1.6836  nodes=nodes
  Pipe_Connection_2 : $bdroot/Storage/Thermal/Storage_Ports/Pipe_Connection  h_in=pipe2inlet  h_out=pipe2outlet  hgt=hgt  dpipe=pipe2dia  dstg=dia  height=0.67344  nodes=nodes
  T_Sensor_Surface : $bdroot/Control/T_Sensor_Surface  pos=Tsensor  tdel=10  t0=mean(tini)
  select_T : Selector  InputPortWidth=nodes  IndexOptions=Index vector (dialog)  Indices=[1 2 3 4 5 6 7 8 9 10]  OutputSizes=1
  sfun_storageTnodes : $bdroot/Basic/Thermal_Models/sfun_storageTnodes  uloss=uwall  ubot=ubot  utop=utop  cond=axcond  volume=volume  dia=dia  standing=standing cylinder  tini=tini  nodes=nodes  nconnect=4  elimthermocline=2  condinvtc=1e5
  Sdat : Outport
  Tsensors : Outport  Port=2
  THB_hx : Outport  Port=3
  THBdhw : Outport  Port=4
  THBcirc : Outport  Port=5
  wires:
  Electric_Heating_1/1 -> sfun_storageTnodes/5
  Pel/1 -> CreateSdat/20, Electric_Heating_1/1  "PelHeater1"
  sfun_storageTnodes/1 -> CreateSdat/2  "Energy"
  HX_EN12977_1/1 -> sfun_storageTnodes/4
  Pipe_Connection_2/2 -> THBcirc/1, CreateSdat/7  "THBoutPipe2"
  Pipe_Connection_2/1 -> sfun_storageTnodes/3
  THB_circ/1 -> CreateSdat/6, Pipe_Connection_2/2, Electric_Heating_1/2  "THBinPipe2"
  Tamb/1 -> sfun_storageTnodes/1, CreateSdat/1  "Tamb"
  select_T/1 -> CreateSdat/3  "Tnodes"
  sfun_storageTnodes/2 -> select_T/1, T_Sensor_Surface/1, HX_EN12977_1/1, Pipe_Connection_2/1, Pipe_Connection_1/1  "Tnodes"
  CreateSdat/1 -> Sdat/1
  THB_dhw/1 -> CreateSdat/4, Pipe_Connection_1/2  "THBinPipe1"
  Pipe_Connection_1/2 -> THBdhw/1, CreateSdat/5  "THBoutPipe1"
  Pipe_Connection_1/1 -> sfun_storageTnodes/2
  THB_HX/1 -> CreateSdat/14, HX_EN12977_1/2
  HX_EN12977_1/2 -> CreateSdat/15, THB_hx/1
  T_Sensor_Surface/1 -> Tsensors/1
  Constant_THB/1 -> CreateSdat/11, CreateSdat/12, CreateSdat/13, CreateSdat/10, CreateSdat/8, CreateSdat/9
  Constant_THB1/1 -> CreateSdat/16, CreateSdat/17, CreateSdat/18, CreateSdat/19

== system carnot/Storage/Thermal/Storage_Type_3 ==
  note: lower heat exchanger (solar)
  note: pipe connection for DHW circulation
  note: pipe connection for DHW
  note: upper heat exchanger (backup heater)
  Tamb : Inport
  THB_HX_up : Inport  Port=2
  THB_HX_low : Inport  Port=3
  THB_dhw : Inport  Port=4
  THB_circ : Inport  Port=5
  Pel : Inport  Port=6
  Constant_THB : $bdroot/Source/Simple/Constant_THB  t=20  mdot=0  p=1e5  mID=No Pressure Drop  fluid=Water  mix=0  mix2=0  mix3=0  dia=0.02  hgt=0
  Constant_THB1 : $bdroot/Source/Simple/Constant_THB  t=20  mdot=0  p=1e5  mID=No Pressure Drop  fluid=Water  mix=0  mix2=0  mix3=0  dia=0.02  hgt=0
  CreateSdat : $bdroot/Basic/Thermal_Models/CreateSdat  volume=volume  stgtype=stgtype
  Electric_Heating_1 : $bdroot/Storage/Thermal/Storage_Ports/Electric_Heating  hin=heater1start  hout=heater1end  nodes=nodes
  HX_EN12977_1 : $bdroot/Storage/Thermal/Storage_Ports/HX_EN12977  h_in=hx1inlet  h_out=hx1outlet  hgt=hgt  dia=hx1dia  height=-0.35368  ua0=hx1uac  uam=hx1uam  uat=hx1uat  uat2=hx1_uat2  dplin=hx1dplin  dpqua=hx1dpqua  nodes=nodes
  HX_EN12977_2 : $bdroot/Storage/Thermal/Storage_Ports/HX_EN12977  h_in=hx2inlet  h_out=hx2outlet  hgt=hgt  dia=hx2dia  height=-0.70736  ua0=hx2uac  uam=hx2uam  uat=hx2uat  uat2=hx2_uat2  dplin=hx2dplin  dpqua=hx2dpqua  nodes=nodes
  Pipe_Connection_1 : $bdroot/Storage/Thermal/Storage_Ports/Pipe_Connection  h_in=pipe1inlet  h_out=pipe1outlet  hgt=hgt  dpipe=pipe1dia  dstg=dia  height=1.7684  nodes=nodes
  Pipe_Connection_2 : $bdroot/Storage/Thermal/Storage_Ports/Pipe_Connection  h_in=pipe2inlet  h_out=pipe2outlet  hgt=hgt  dpipe=pipe2dia  dstg=dia  height=0.70736  nodes=nodes
  T_Sensor_Surface : $bdroot/Control/T_Sensor_Surface  pos=Tsensor  tdel=10  t0=mean(tini)
  select_T : Selector  InputPortWidth=nodes  IndexOptions=Index vector (dialog)  Indices=[1 2 3 4 5 6 7 8 9 10]  OutputSizes=1
  sfun_storageTnodes : $bdroot/Basic/Thermal_Models/sfun_storageTnodes  uloss=uwall  ubot=ubot  utop=utop  cond=axcond  volume=volume  dia=dia  standing=standing cylinder  tini=tini  nodes=nodes  nconnect=5  elimthermocline=2  condinvtc=1e5
  Sdat : Outport
  Tsensors : Outport  Port=2
  THB_hx_up : Outport  Port=3
  THB_hx_low : Outport  Port=4
  THBdhw : Outport  Port=5
  THBcirc : Outport  Port=6
  wires:
  Electric_Heating_1/1 -> sfun_storageTnodes/6
  Pel/1 -> CreateSdat/20, Electric_Heating_1/1  "PelHeater1"
  T_Sensor_Surface/1 -> Tsensors/1
  HX_EN12977_1/2 -> CreateSdat/15, THB_hx_up/1  "THBoutHX1"
  THB_HX_up/1 -> CreateSdat/14, HX_EN12977_1/2  "THBinHX1"
  Pipe_Connection_1/1 -> sfun_storageTnodes/3
  Pipe_Connection_1/2 -> THBdhw/1, CreateSdat/5  "THBoutPipe1"
  THB_dhw/1 -> CreateSdat/4, Pipe_Connection_1/2  "THBinPipe1"
  CreateSdat/1 -> Sdat/1
  sfun_storageTnodes/2 -> Pipe_Connection_2/1, Pipe_Connection_1/1, HX_EN12977_2/1, HX_EN12977_1/1, T_Sensor_Surface/1, select_T/1  "Tnodes"
  select_T/1 -> CreateSdat/3  "Tnodes"
  HX_EN12977_2/1 -> sfun_storageTnodes/2
  HX_EN12977_2/2 -> CreateSdat/17, THB_hx_low/1  "THBoutHX2"
  THB_HX_low/1 -> CreateSdat/16, HX_EN12977_2/2  "THBinHX2"
  Tamb/1 -> sfun_storageTnodes/1, CreateSdat/1  "Tamb"
  THB_circ/1 -> CreateSdat/6, Pipe_Connection_2/2, Electric_Heating_1/2  "THBinPipe2"
  Pipe_Connection_2/1 -> sfun_storageTnodes/4
  Pipe_Connection_2/2 -> THBcirc/1, CreateSdat/7  "THBoutPipe2"
  HX_EN12977_1/1 -> sfun_storageTnodes/5
  sfun_storageTnodes/1 -> CreateSdat/2  "Energy"
  Constant_THB1/1 -> CreateSdat/18, CreateSdat/19
  Constant_THB/1 -> CreateSdat/10, CreateSdat/11, CreateSdat/12, CreateSdat/13, CreateSdat/8, CreateSdat/9

== system carnot/Storage/Thermal/Storage_Type_4 ==
  note: heat exchanger for DHW circulation
  note: heat exchanger solar
  note: pipe connection for house heating
  note: pipe connection to charge DHW section
  note: Domestic hot water heat exchanger
  Tamb : Inport
  THB_dhw : Inport  Port=2
  THB_chg_up : Inport  Port=3
  THB_dis_mid : Inport  Port=4
  THB_hx_low : Inport  Port=5
  THB_circ : Inport  Port=6
  Pel : Inport  Port=7
  Constant_THB : $bdroot/Source/Simple/Constant_THB  t=20  mdot=0  p=1e5  mID=No Pressure Drop  fluid=Water  mix=0  mix2=0  mix3=0  dia=0.02  hgt=0
  Constant_THB1 : $bdroot/Source/Simple/Constant_THB  t=20  mdot=0  p=1e5  mID=No Pressure Drop  fluid=Water  mix=0  mix2=0  mix3=0  dia=0.02  hgt=0
  CreateSdat : $bdroot/Basic/Thermal_Models/CreateSdat  volume=volume  stgtype=stgtype
  Electric_Heating : $bdroot/Storage/Thermal/Storage_Ports/Electric_Heating  hin=heater1start  hout=heater1end  nodes=nodes
  HX_EN12977_1 : $bdroot/Storage/Thermal/Storage_Ports/HX_EN12977  h_in=hx1inlet  h_out=hx1outlet  hgt=hgt  dia=hx1dia  height=-0.72432  ua0=hx1uac  uam=hx1uam  uat=hx1uat  uat2=hx1_uat2  dplin=hx1dplin  dpqua=hx1dpqua  nodes=nodes
  HX_EN12977_2 : $bdroot/Storage/Thermal/Storage_Ports/HX_EN12977  h_in=hx2inlet  h_out=hx2outlet  hgt=hgt  dia=hx2dia  height=1.8108  ua0=hx2uac  uam=hx2uam  uat=hx2uat  uat2=hx2_uat2  dplin=hx2dplin  dpqua=hx2dpqua  nodes=nodes
  HX_EN12977_3 : $bdroot/Storage/Thermal/Storage_Ports/HX_EN12977  h_in=hx3inlet  h_out=hx3outlet  hgt=hgt  dia=hx3dia  height=0.18108  ua0=hx3uac  uam=hx3uam  uat=hx3uat  uat2=uat2  dplin=hx3dplin  dpqua=hx3dpqua  nodes=nodes
  Pipe_Connection_2 : $bdroot/Storage/Thermal/Storage_Ports/Pipe_Connection  h_in=pipe2inlet  h_out=pipe2outlet  hgt=hgt  dpipe=pipe2dia  dstg=dia  height=0.18108  nodes=nodes
  Pipe_Connection_3 : $bdroot/Storage/Thermal/Storage_Ports/Pipe_Connection  h_in=pipe3inlet  h_out=pipe3outlet  hgt=hgt  dpipe=pipe3dia  dstg=dia  height=-0.72432  nodes=nodes
  T_Sensor_Surface : $bdroot/Control/T_Sensor_Surface  pos=Tsensor  tdel=10  t0=mean(tini)
  select_T : Selector  InputPortWidth=nodes  IndexOptions=Index vector (dialog)  Indices=[1 3 5 7 9 11 13 15 17 19]  OutputSizes=1
  sfun_storageTnodes : $bdroot/Basic/Thermal_Models/sfun_storageTnodes  uloss=uwall  ubot=ubot  utop=utop  cond=axcond  volume=volume  dia=dia  standing=standing cylinder  tini=tini  nodes=nodes  nconnect=6  elimthermocline=2  condinvtc=1e5
  Sdat : Outport
  Tsensors : Outport  Port=2
  THBdhw : Outport  Port=3
  THBchg_up : Outport  Port=4
  THBdis_mid : Outport  Port=5
  THBhx_low : Outport  Port=6
  THBcirc : Outport  Port=7
  wires:
  Electric_Heating/1 -> sfun_storageTnodes/7
  Pel/1 -> CreateSdat/20, Electric_Heating/1
  sfun_storageTnodes/1 -> CreateSdat/2  "Energy"
  HX_EN12977_1/1 -> sfun_storageTnodes/5
  Pipe_Connection_2/2 -> THBdis_mid/1, CreateSdat/7  "THBoutPipe2"
  Pipe_Connection_2/1 -> sfun_storageTnodes/4
  THB_dis_mid/1 -> CreateSdat/6, Pipe_Connection_2/2, Electric_Heating/2  "THBinPipe2"
  Tamb/1 -> sfun_storageTnodes/1, CreateSdat/1  "Tamb"
  THB_dhw/1 -> CreateSdat/16, HX_EN12977_2/2  "THBinHX2"
  HX_EN12977_2/2 -> CreateSdat/17, THBdhw/1  "THBoutHX2"
  HX_EN12977_2/1 -> sfun_storageTnodes/2
  select_T/1 -> CreateSdat/3  "Tnodes"
  sfun_storageTnodes/2 -> select_T/1, T_Sensor_Surface/1, Pipe_Connection_2/1, HX_EN12977_3/1, HX_EN12977_1/1, Pipe_Connection_3/1, HX_EN12977_2/1  "Tnodes"
  CreateSdat/1 -> Sdat/1
  THB_chg_up/1 -> CreateSdat/8, Pipe_Connection_3/2  "THBinPipe3"
  Pipe_Connection_3/2 -> THBchg_up/1, CreateSdat/9  "THBoutPipe3"
  Pipe_Connection_3/1 -> sfun_storageTnodes/3
  THB_hx_low/1 -> CreateSdat/14, HX_EN12977_1/2  "THBinHX1"
  HX_EN12977_1/2 -> CreateSdat/15, THBhx_low/1  "THBoutHX1"
  T_Sensor_Surface/1 -> Tsensors/1
  THB_circ/1 -> CreateSdat/18, HX_EN12977_3/2  "THBinHX3"
  HX_EN12977_3/1 -> sfun_storageTnodes/6
  HX_EN12977_3/2 -> CreateSdat/19, THBcirc/1  "THBoutHX3"
  Constant_THB/1 -> CreateSdat/5, CreateSdat/4
  Constant_THB1/1 -> CreateSdat/12, CreateSdat/13, CreateSdat/11, CreateSdat/10
